simulink model "emulacion_planta"  (R2020b)
settings: Solver=VariableStepAuto  StartTime=0.0  StopTime=inf  FixedStep=Ts  RelTol=1e-3
libraries: instrumentlib x2
settings Model: Creator=Acer  LastModifiedBy=Acer

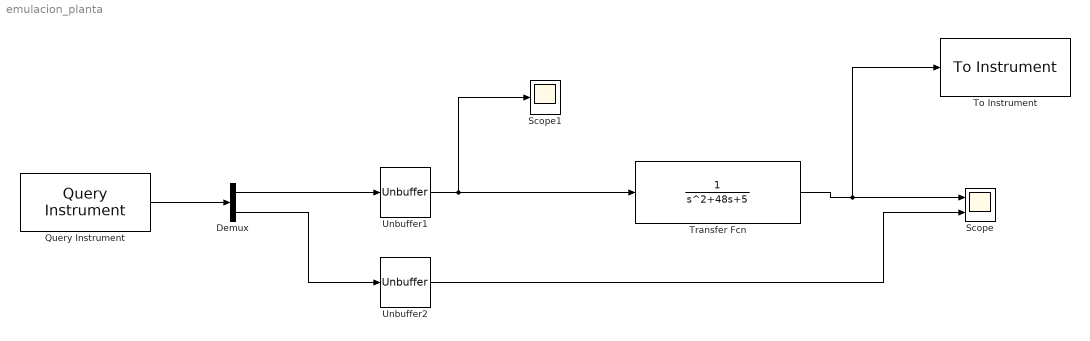
== system emulacion_planta ==
  Demux : Demux  Outputs=2
  Query Instrument : instrumentlib/Query Instrument  sampleTime=Ts  isWorkspaceObject=off  timeout=10  inputBufferSize=512  protocol=Serial  serialPort=COM3  baudRate=115200  gpibVendor=Keysight Technologies  boardIndex=0  primaryAddress=1  secondaryAddress=0  visaVendor=Keysight  visaSerialPort=0  chassisIndex=0  logicalAddress=0  tcpRemoteHost='127.0.0.1'  tcpRemotePort=4500  udpRemoteHost='127.0.0.1'  udpRemotePort=9090  visaTCPBoardIndex=0  visaTCPRemoteHost='127.0.0.1'  usbBoardIndex=0  usbManufID=0  usbModelCode=0  usbSerialNumber=0  initAction=None  initCommand='DATA:SOURCE CH1'  initFunction=get  queryCommand=''  responseFormat=ASCII  asciiFormatting='%f,%f\n'  precision=8-bit integer  byteOrder=Little endian  valuesToRead=1  removeBytes=on  afterOutputAction=Repeat query for new data  enableFrames=on  frameSize=2
      settings: SourceProductBaseCode=IC
  Scope : Scope  NumInputPorts=2
  Scope1 : Scope
  To Instrument : instrumentlib/To Instrument  sampleTime=-1  isWorkspaceObject=off  timeout=10  inputBufferSize=8192  protocol=Serial  serialPort=COM3  baudRate=115200  gpibVendor=ICS Electronics  boardIndex=0  primaryAddress=1  secondaryAddress=0  visaVendor=Keysight  visaSerialPort=0  chassisIndex=0  logicalAddress=0  tcpRemoteHost='127.0.0.1'  tcpRemotePort=4500  udpRemoteHost='127.0.0.1'  udpRemotePort=9090  visaTCPBoardIndex=0  visaTCPRemoteHost='127.0.0.1'  usbBoardIndex=0  usbManufID=0  usbModelCode=0  usbSerialNumber=0  initAction=None  initCommand='DATA:SOURCE CH1'  initFunction=get  command=''  sendFormat=ASCII  asciiFormatting='%5.2f\n'  precision=8-bit integer  byteOrder=Little endian
      settings: SourceProductBaseCode=IC
  Transfer Fcn : TransferFcn  Denominator=[1 48 5]
  Unbuffer1 : Unbuffer
  Unbuffer2 : Unbuffer
  wires:
  Transfer Fcn/1 -> To Instrument/1, Scope/1
  Query Instrument/1 -> Demux/1
  Demux/1 -> Unbuffer1/1
  Demux/2 -> Unbuffer2/1
  Unbuffer2/1 -> Scope/2
  Unbuffer1/1 -> Transfer Fcn/1, Scope1/1
